simulink model "sa_vjezbi"  (R2017b)
settings: Solver=VariableStepAuto  StartTime=0.0  StopTime=100  RelTol=1e-3
libraries: simulink x10
settings Model: Creator=DT User  LastModifiedBy=DT User

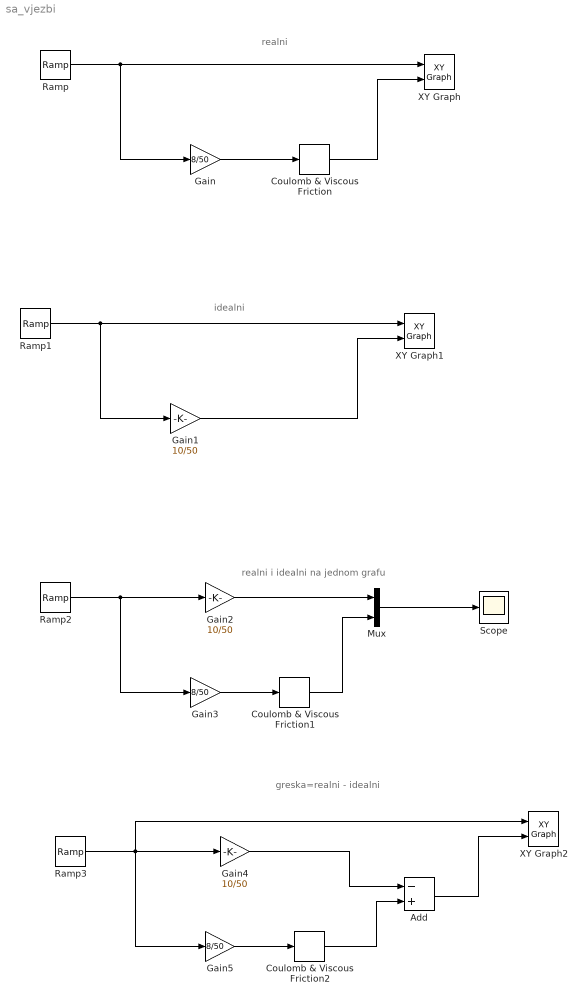
== system sa_vjezbi ==
  note: realni
  note: idealni
  note: realni i idealni na jednom grafu
  note: greska=realni - idealni
  Add : Sum  Inputs=-+
  Coulomb & Viscous Friction : simulink/Discontinuities/Coulomb & Viscous Friction  offset=2  gain=1
      settings: SourceProductName=Simulink
  Coulomb & Viscous Friction1 : simulink/Discontinuities/Coulomb & Viscous Friction  offset=2  gain=1
      settings: SourceProductName=Simulink
  Coulomb & Viscous Friction2 : simulink/Discontinuities/Coulomb & Viscous Friction  offset=2  gain=1
      settings: SourceProductName=Simulink
  Gain : Gain  Gain=8/50
  Gain1 : Gain  Gain=10/50
  Gain2 : Gain  Gain=10/50
  Gain3 : Gain  Gain=8/50
  Gain4 : Gain  Gain=10/50
  Gain5 : Gain  Gain=8/50
  Mux : Mux  Inputs=2
  Ramp{,1..3} (4 alike) : simulink/Sources/Ramp  slope=1  start=0  X0=-50
  Scope : Scope
  XY Graph : simulink/Sinks/XY Graph  xmin=-50  xmax=50  ymin=-10  ymax=10  st=-1
  XY Graph1 : simulink/Sinks/XY Graph  xmin=-50  xmax=50  ymin=-10  ymax=10  st=-1
  XY Graph2 : simulink/Sinks/XY Graph  xmin=-50  xmax=50  ymin=-10  ymax=10  st=-1
  wires:
  Gain/1 -> Coulomb & Viscous Friction/1
  Coulomb & Viscous Friction/1 -> XY Graph/2
  Ramp/1 -> Gain/1, XY Graph/1
  Ramp1/1 -> XY Graph1/1, Gain1/1
  Gain1/1 -> XY Graph1/2
  Ramp2/1 -> Gain3/1, Gain2/1
  Mux/1 -> Scope/1
  Gain3/1 -> Coulomb & Viscous Friction1/1
  Coulomb & Viscous Friction1/1 -> Mux/2
  Gain2/1 -> Mux/1
  Gain4/1 -> Add/1
  Gain5/1 -> Coulomb & Viscous Friction2/1
  Ramp3/1 -> XY Graph2/1, Gain4/1, Gain5/1
  Coulomb & Viscous Friction2/1 -> Add/2
  Add/1 -> XY Graph2/2
